simulink model "model"  (R2015a)
settings: Solver=FixedStepDiscrete  StartTime=0.0  StopTime=20  RelTol=1e-3
values from neighbouring files (symbols this model uses):
  Nbar = 0    [teste_integrador.m]
undefined symbols (not defined in the file or in its folder): T
settings Model: Creator=Paul  LastModifiedBy=hdplsa

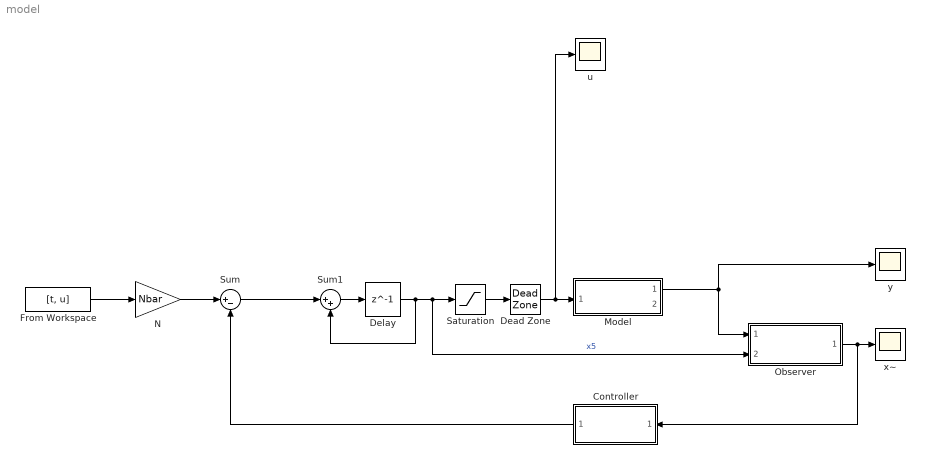
== system model ==
  Controller : ModelReference  ModelNameDialog=controller.slx  SimulationMode=Normal  ModelReferenceVersion=1.3  CopyOfModelName=controller.slx  DefaultDataLogging=on
  Dead Zone : DeadZone  LowerValue=-0.17  UpperValue=0.45  SaturateOnIntegerOverflow=on
  Delay : Delay  DelayLength=1  InitialCondition=0
  From Workspace : FromWorkspace  VariableName=[t, u]  SampleTime=T
  Model : ModelReference  ModelNameDialog=plant.slx  SimulationMode=Normal  ModelReferenceVersion=1.20  CopyOfModelName=plant.slx  DefaultDataLogging=on
  N : Gain  Gain=Nbar
  Observer : ModelReference  ModelNameDialog=observer.slx  SimulationMode=Normal  ModelReferenceVersion=1.5  CopyOfModelName=observer.slx  DefaultDataLogging=on
  Saturation : Saturate  UpperLimit=5  LowerLimit=-5
  Sum : Sum  Inputs=|+-
  Sum1 : Sum  Inputs=|++
  u : Scope
      settings: TimeRange=20  YMin=-1000  YMax=0  SaveName=ScopeData2
  x~ : Scope
      settings: TimeRange=20  YMin=-1000  YMax=0
  y : Scope
      settings: TimeRange=20  YMin=-1000  YMax=0
  wires:
  Model/1 -> y/1, Observer/1
  Observer/1 -> x~/1, Controller/1
  N/1 -> Sum/1
  From Workspace/1 -> N/1
  Controller/1 -> Sum/2
  Saturation/1 -> Dead Zone/1
  Delay/1 -> Sum1/2, Observer/2, Saturation/1  "x5"
  Sum1/1 -> Delay/1
  Dead Zone/1 -> u/1, Model/1
  Sum/1 -> Sum1/1
